simulink model "untitled1"  (R2019a)
settings: Solver=VariableStepAuto  StartTime=0.0  StopTime=10.0  RelTol=1e-3
settings Model: Creator=JanAriel  LastModifiedBy=JanAriel

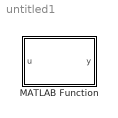
== system untitled1 ==
  MATLAB Function : MATLAB Function  TreatAsAtomicUnit=on

== matlab function untitled1/MATLAB Function ==
  data: u input; y output
function y = fcn(u)
%#codegen

m1 = 5;
m2 = 5;

lc1 = (0.7/2);
lc2 = (0.7/2);

l1 = 0.7;
l2 = 0.7;

r1 = 0.05;
r2 = 0.05;

d_1 = 0.15



alpha =[0 0];
d = [d_1 0];
% theta = [q1 q2];
theta = u;
a = [a1 a2];

% A = [cos(theta(i)) -cos(alpha(i))*sin(theta(i)) sin(alpha(i))*sin(theta(i)) a(i)*cos(theta(i));
%         sin(theta(i)) cos(alpha(i))*cos(theta(i)) -sin(alpha(i))*cos(theta(i)) a(i)*sin(theta(i));
%         0 sin(alpha(i)) cos(alpha(i)) d(i);
%         0 0 0 1]
    
collect = [];
T = eye(4);

for i = 1:2
    collect{i} = [cos(theta(i)) -cos(alpha(i))*sin(theta(i)) sin(alpha(i))*sin(theta(i)) a(i)*cos(theta(i));
        sin(theta(i)) cos(alpha(i))*cos(theta(i)) -sin(alpha(i))*cos(theta(i)) a(i)*sin(theta(i));
        0 sin(alpha(i)) cos(alpha(i)) d(i);
        0 0 0 1];   
    T = T* collect{i};
end
A1 = collect{1};
A2 = collect{2};
A1c = subs(A1, [a1,a2],[l1,l2]);

R1 = A1(1:3,1:3)
R2 = A2(1:3,1:3)

J1 = [cross([0 0 1]',T(1:3,4)); [0 0 1]'];
J2 = [cross(A1(1:3,3),T(1:3,4)-A1(1:3,4)) ; A1(1:3,3)];


% Setup
J1_v = [cross([0 0 1]',A1(1:3,4))];
J1_w = [0 0 1]';
J2_v = [cross(A1c(1:3,3),T(1:3,4)-A1c(1:3,4))];
J2_w = [A1c(1:3,3)];


% Collect
J1v = [J1_v zeros(3,1)];
J1w = [J1_w zeros(3,1)];

% Collect
J1_v = [cross([0 0 1]',A1c(1:3,4))];
J2v = [(J1_v+J2_v) J2_v];
J2w = [(J2_v+J2_v) J2_v];

% Substitute
J1c_v = subs(J1v,[a1,a2],[lc1,lc2]);
J1c_w = subs(J1w,[a1,a2],[lc1,lc2]);
J2c_v = subs(J2v , [a1,a2],[lc1,lc2]);
J2c_w = subs(J2w , [a1,a2],[lc1,lc2]);


J = simplify([J1 J2]);

I_2 = (1/12)*m1*(3*r1^2 + l1^2);
I_2yy = (1/2)*m1*r1^2;

I_3 = (1/12)*m2*(3*r2^2 + l2^2);
I_3yy = (1/2)*m2*r2^2;

I2res = I_2 - I_2yy;
I3res = I_3 - I_3yy;


I_col = (J1c_w' * R1 * I2res * R1' * J1c_w + J2c_w' * R2 * I3res * R2' * J2c_w)
D = m1*(J1c_v')*J1c_v + m2*(J2c_v') * J2c_v + I_col;
Dq = simplify(D);

y = u;
